simulink model "ship2021a"  (R2021a)
settings: Solver=VariableStepAuto  StartTime=0.0  StopTime=1500  RelTol=1e-3
undefined symbols (not defined in the file): D, Dn, M, surge_lambda, surge_omega_n, surge_zeta
libraries: mssSimulink x3, simulink x1
settings Model: Creator=simengangstad  LastModifiedBy=simengangstad

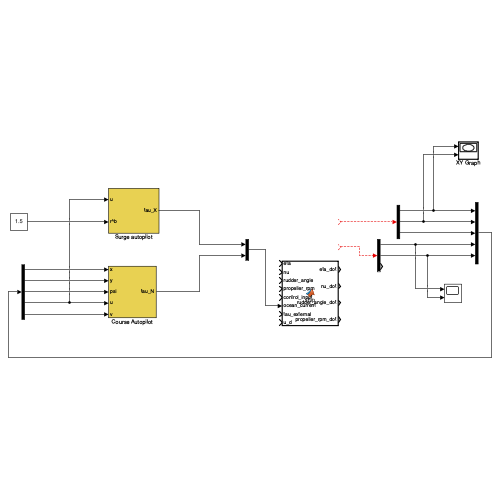
[thumbnail: Simulink's stored preview of the top-level diagram]
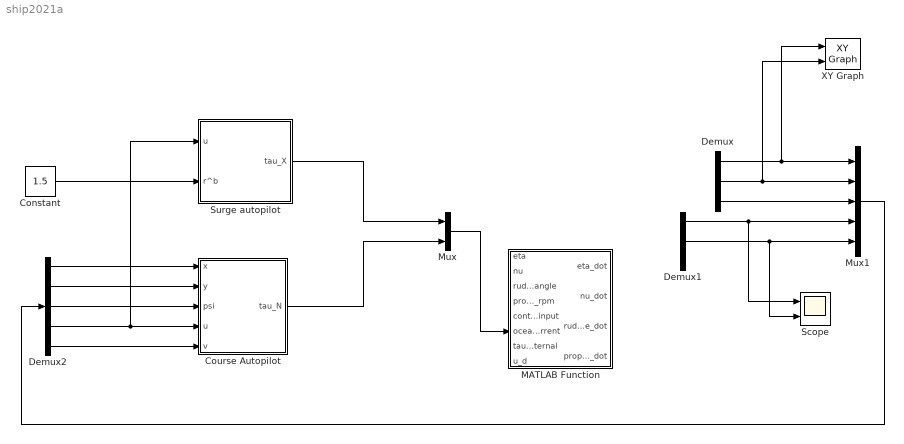
== system ship2021a ==
  Constant : Constant  Value=1.5
  Course Autopilot : Subsystem
  Demux : Demux  Outputs=3
  Demux1 : Demux  Outputs=3
  Demux2 : Demux  Outputs=5
  MATLAB Function : MATLAB Function  TreatAsAtomicUnit=on
  Mux : Mux  Inputs=2
  Mux1 : Mux  Inputs=5
  Scope : Scope  NumInputPorts=2
  Surge autopilot : Subsystem
  XY Graph : simulink/Sinks/XY Graph  xmin=-1  xmax=1  ymin=-1  ymax=1  st=-1
  wires:
  ? -> Demux1/1
  ? -> Demux/1
  Demux/2 -> XY Graph/2, Mux1/2
  Demux1/1 -> Scope/1, Mux1/4
  Constant/1 -> Surge autopilot/2(r^b)
  Surge autopilot/1(tau_X) -> Mux/1
  Demux/1 -> XY Graph/1, Mux1/1
  Demux/3 -> Mux1/3
  Demux1/2 -> Scope/2, Mux1/5
  Demux2/1 -> Course Autopilot/1(x)
  Demux2/2 -> Course Autopilot/2(y)
  Demux2/3 -> Course Autopilot/3(psi)
  Demux2/4 -> Surge autopilot/1(u), Course Autopilot/4(u)
  Demux2/5 -> Course Autopilot/5(v)
  Mux1/1 -> Demux2/1
  Course Autopilot/1(tau_N) -> Mux/2
  Mux/1 -> MATLAB Function/6(ocean_current)

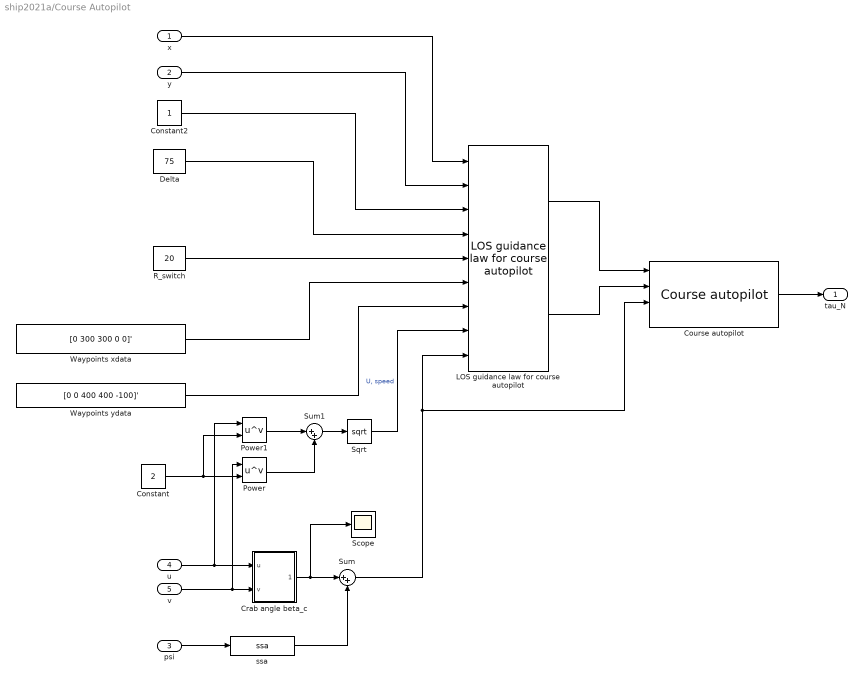
== system ship2021a/Course Autopilot ==
  x : Inport
  y : Inport  Port=2
  psi : Inport  Port=3
  u : Inport  Port=4
  v : Inport  Port=5
  Constant : Constant  Value=2
  Constant2 : Constant
  Course autopilot : mssSimulink/Control/Autopilots/Course autopilot  wn=yaw_omega_n  zeta=1  T_nomoto=yaw_T  m=M(3, 3)
  Crab angle beta_c : Subsystem
  Delta : Constant  Value=75
  LOS guidance law for course autopilot : mssSimulink/Guidance/LOS guidance law for course autopilot  SystemSampleTime=-1  VariantActivationTime=update diagram  Latency=0  AutoFrameSizeCalculation=off
  Power : Math  Operator=pow  SaturateOnIntegerOverflow=on
  Power1 : Math  Operator=pow  SaturateOnIntegerOverflow=on
  R_switch : Constant  Value=20
  Scope : Scope
  Sqrt : Sqrt  SaturateOnIntegerOverflow=on
  Sum : Sum  Inputs=|++
  Sum1 : Sum  Inputs=|++
  Waypoints xdata : Constant  Value=[0 300 300 0 0]'
  Waypoints ydata : Constant  Value=[0 0 400 400 -100]'
  "ssa   " : mssSimulink/Utilities/Math Operations/ssa  SystemSampleTime=-1  VariantActivationTime=update diagram  Latency=0  AutoFrameSizeCalculation=off
  tau_N : Outport
  wires:
  Sqrt/1 -> LOS guidance law for course autopilot/8  "U, speed"
  Course autopilot/1 -> tau_N/1
  x/1 -> LOS guidance law for course autopilot/1
  Delta/1 -> LOS guidance law for course autopilot/4
  y/1 -> LOS guidance law for course autopilot/2
  Sum/1 -> LOS guidance law for course autopilot/9, Course autopilot/3
  Constant2/1 -> LOS guidance law for course autopilot/3
  Waypoints xdata/1 -> LOS guidance law for course autopilot/6
  Waypoints ydata/1 -> LOS guidance law for course autopilot/7
  LOS guidance law for course autopilot/1 -> Course autopilot/1
  LOS guidance law for course autopilot/2 -> Course autopilot/2
  R_switch/1 -> LOS guidance law for course autopilot/5
  u/1 -> Crab angle beta_c/1(u), Power1/1
  v/1 -> Power/1, Crab angle beta_c/2(v)
  psi/1 -> "ssa   "/1
  Crab angle beta_c/1(beta_c) -> Scope/1, Sum/1
  "ssa   "/1 -> Sum/2
  Constant/1 -> Power1/2, Power/2
  Power1/1 -> Sum1/1
  Power/1 -> Sum1/2
  Sum1/1 -> Sqrt/1

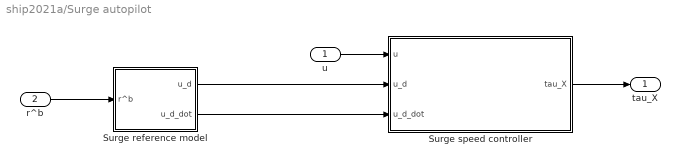
== system ship2021a/Surge autopilot ==
  u : Inport
  r^b : Inport  Port=2
  Surge reference model : Subsystem
  Surge speed controller : Subsystem
  tau_X : Outport
  wires:
  u/1 -> Surge speed controller/1(u)
  Surge reference model/1(u_d) -> Surge speed controller/2("u_d ")
  Surge speed controller/1(tau_X) -> tau_X/1
  Surge reference model/2(u_d_dot) -> Surge speed controller/3("u_d_dot ")
  r^b/1 -> Surge reference model/1(r^b)

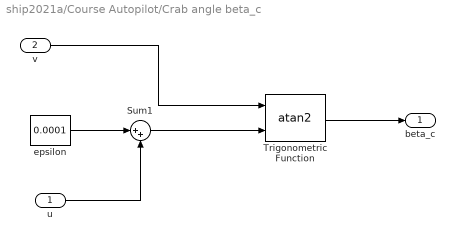
== system ship2021a/Course Autopilot/Crab angle beta_c ==
  u : Inport
  v : Inport  Port=2
  Sum1 : Sum  Inputs=|++  InputSameDT=on  SaturateOnIntegerOverflow=on  OutDataTypeStr=Inherit: Same as first input
  Trigonometric Function : Trigonometry  Operator=atan2
  epsilon : Constant  Value=0.0001
  beta_c : Outport
  wires:
  Trigonometric Function/1 -> beta_c/1
  v/1 -> Trigonometric Function/1
  Sum1/1 -> Trigonometric Function/2
  u/1 -> Sum1/2
  epsilon/1 -> Sum1/1

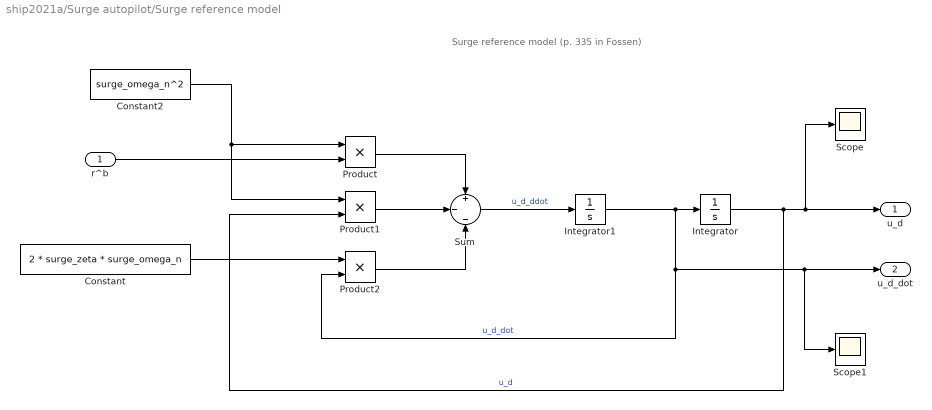
== system ship2021a/Surge autopilot/Surge reference model ==
  note: Surge reference model (p. 335 in Fossen)
  r^b : Inport
  Constant : Constant  Value=2 * surge_zeta * surge_omega_n
  Constant2 : Constant  Value=surge_omega_n^2
  Integrator : Integrator
  Integrator1 : Integrator
  Product : Product
  Product1 : Product
  Product2 : Product
  Scope : Scope
  Scope1 : Scope
  Sum : Sum  Inputs=+|-|-
  u_d : Outport
  u_d_dot : Outport  Port=2
  wires:
  r^b/1 -> Product/2
  Product2/1 -> Sum/3
  Product/1 -> Sum/1
  Constant/1 -> Product2/1
  Sum/1 -> Integrator1/1  "u_d_ddot"
  Constant2/1 -> Product/1, Product1/1
  Product1/1 -> Sum/2
  Integrator/1 -> Scope/1, u_d/1, Product1/2  "u_d"
  Integrator1/1 -> u_d_dot/1, Scope1/1, Product2/2, Integrator/1  "u_d_dot"

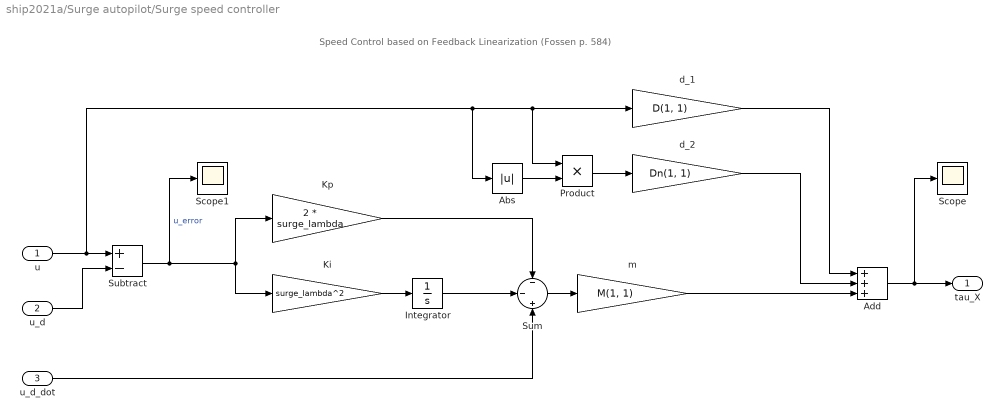
== system ship2021a/Surge autopilot/Surge speed controller ==
  note: Speed Control based on Feedback Linearization (Fossen p. 584)
  u : Inport
  "u_d " : Inport  Port=2
  "u_d_dot " : Inport  Port=3
  Abs : Abs
  Add : Sum  Inputs=+++
  Integrator : Integrator
  Ki : Gain  Gain=surge_lambda^2  SaturateOnIntegerOverflow=on  OutDataTypeStr=Inherit: Same as input  ParamDataTypeStr=Inherit: Same as input
  Kp : Gain  Gain=2 * surge_lambda  SaturateOnIntegerOverflow=on  OutDataTypeStr=Inherit: Same as input  ParamDataTypeStr=Inherit: Same as input
  Product : Product
  Scope : Scope
  Scope1 : Scope
  Subtract : Sum  Inputs=+-
  Sum : Sum  Inputs=-|-|+
  d_1 : Gain  Gain=D(1, 1)  SaturateOnIntegerOverflow=on  OutDataTypeStr=Inherit: Same as input  ParamDataTypeStr=Inherit: Same as input
  d_2 : Gain  Gain=Dn(1, 1)  SaturateOnIntegerOverflow=on  OutDataTypeStr=Inherit: Same as input  ParamDataTypeStr=Inherit: Same as input
  m : Gain  Gain=M(1, 1)  SaturateOnIntegerOverflow=on  OutDataTypeStr=Inherit: Same as input  ParamDataTypeStr=Inherit: Same as input
  tau_X : Outport
  wires:
  d_2/1 -> Add/2
  Product/1 -> d_2/1
  Ki/1 -> Integrator/1
  Sum/1 -> m/1
  Abs/1 -> Product/2
  Integrator/1 -> Sum/2
  u/1 -> Abs/1, Product/1, d_1/1, Subtract/1
  m/1 -> Add/3
  d_1/1 -> Add/1
  Add/1 -> Scope/1, tau_X/1
  Kp/1 -> Sum/1
  "u_d "/1 -> Subtract/2
  "u_d_dot "/1 -> Sum/3
  Subtract/1 -> Scope1/1, Ki/1, Kp/1  "u_error"

== matlab function ship2021a/MATLAB Function ==
  data: eta input; nu input; rudder_angle input; propeller_rpm input; control_input input; eta_dot output; nu_dot output; rudder_angle_dot output; propeller_rpm_dot output; ocean_current input; tau_external input; u_d input
function [eta_dot, nu_dot, rudder_angle_dot, propeller_rpm_dot] = ship(eta, nu, rudder_angle, propeller_rpm, control_input, ocean_current, tau_external, u_d)
%
% returns the time derivative of the state vector: 
% 
% eta   = [x y psi]
% nu    = [u v r]
% delta = actual rudder angle               (rad)
% n     = actual shaft velocity             (rpm)
% 
% The input vector is :
%
% u       = [ delta_c  n_c ]'  where
%
% delta_c = commanded rudder angle          (rad)
% n_c     = commanded shaft velocity        (rpm)
%
% The ocean current vector is: 
%
% nu_c    = [ u_c v_c 0 ]'  where
%
% uc = current velocity in surge            (m/s)
% vc = current velocity in sway             (m/s)
%
% The external environmental force vector is denoted by tau_ext


% Check of input and state dimensions
if length(x) ~= 8
    error('x-vector must have dimension 8 !');
end

if length(u) ~= 2
    error('u-vector must have dimension 2 !');
end

% Dimensional states and input
delta_c = u(1); 
n_c     = u(2);

nu      = x(1:3);
eta     = x(4:6);
delta   = x(7);
n       = x(8); 


nu_r = nu - nu_c;       % Relative velocity
uc = nu_c(1);
vc = nu_c(2);


% Parameters 
m   = 17.0677e6;         % Total mass (kg)
Iz  = 2.1732e10;         % Yaw moment of inertia (kg m^2)
xg  = -3.7;              % CG x-ccordinate (m)
L   = 161;               % length (m)
B   = 21.8;              % beam (m)
T   = 8.9;               % draft (m)
KT  = 0.6367;            % propeller coefficient (-)
KQ  = 0.1390;
Dia = 3.3;               % propeller diameter (m)
rho = 1025;              % density of water (m/s^3)

% Propeller parameters
I_m = 100000;            % Inertia of the rotating parts including the propeller
                         % and added inertia of the water (kgm^2)
T_m = 10;                

% Rudder limitations
delta_max  = 40 * pi/180;        % max rudder angle      (rad)
Ddelta_max = 5  * pi/180;        % max rudder derivative (rad/s)

% Added mass matrix
Xudot = -8.9830e5;
Yvdot = -5.1996e6;
Yrdot =  9.3677e5;
Nvdot =  Yrdot;
Nrdot = -2.4283e10;
MA = -[ Xudot 0 0; 0 Yvdot Yrdot; 0 Nvdot Nrdot ];   % Added mass matrix

% Rigid-body mass matrix
MRB = [ m 0      0 
        0 m      m * xg
        0 m * xg Iz ];        
Minv = inv(MRB + MA);       

% Rudder coefficients
b = 2;
AR = 8;
CB = 0.8;

lambda = b^2 / AR;
tR = 0.45 - 0.28*CB;
CN = 6.13 * lambda / (lambda + 2.25);
aH = 0.75;
xH = -0.4 * L;
xR = -0.5 * L;

% Input matrix
t_thr = 0.05;                                        % Thrust deduction number
X_delta2 = 0.5 * (1 - tR) * rho * AR * CN;           % Rudder coefficients
Y_delta = 0.25 * (1 + aH) * rho * AR * CN; 
N_delta = 0.25 * (xR + aH * xH) * rho * AR * CN;   

Bi = @(u_r,delta) [ (1-t_thr)  -u_r^2 * X_delta2 * delta
                        0      -u_r^2 * Y_delta
                        0      -u_r^2 * N_delta            ];
    
% State-dependent time-varying matrices

% Restoring force for rigid-body
CRB = m * nu_r(3) * [ 0 -1 -xg 
                      1  0  0 
                      xg 0  0  ];         

% Restoring force for added mass 
CA = [0 0 Yvdot * nu_r(2) + Yrdot * nu_r(3); 
      0 0 -Xudot * nu_r(1); 
      -Yvdot * nu_r(2) - Yrdot * nu_r(3) Xudot * nu_r(1) 0];    

% Linear damping
T1 = 20; T2 = 20; T6 = 10;      % Natural Period for Surge, Sway and Yaw (s)
Xu = -(m-Xudot) / T1;
Yv = -(m-Yvdot) / T2;
Nr = -(Iz-Nrdot) / T6;
D = -diag([Xu Yv Nr]); 

% Nonlinear surge damping
eps = 0.001;
CR = 0;
k = 0.1;
S = B*L + 2*T*(B+L);
v = 1e-6;
Rn = L / v * abs(nu_r(1));
Cf = 0.075 / (log10(Rn) - 2 + eps)^2 + CR;
Xns = -0.5 * rho * S * (1+k) * Cf * abs(nu_r(1)) * nu_r(1);

% Nonlinear cross-flow drag
Cd_2d = Hoerner(B,T);
dx = L/10;
Ycf = 0; Ncf = 0;
for xL = -L/2:dx:L/2
    Ucf = abs(nu_r(2) + xL * nu_r(3)) * (nu_r(2) + xL * nu_r(3));
    Ycf = Ycf - 0.5 * rho * T * Cd_2d * Ucf * dx;
    Ncf = Ncf - 0.5 * rho * T * Cd_2d * xL * Ucf * dx;
end
d = -[Xns Ycf Ncf]';

% Thrust
thr = rho * Dia^4 * KT * abs(n) * n;

% Ship dynamics
R = Rzyx(0, 0, eta(3));
u = [ thr delta ]';
tau = Bi(nu_r(1), delta) * u;

nu_dot = [nu(3) * vc -nu(3) * uc 0]' + Minv * (tau_ext + tau - (CRB + CA + D) * nu_r - d);
eta_dot = R * nu;    

% Rudder saturation and dynamics
if abs(delta_c) >= delta_max
    delta_c = sign(delta_c)*delta_max;
end

delta_dot = delta_c - delta;
if abs(delta_dot) >= Ddelta_max
    delta_dot = sign(delta_dot)*Ddelta_max;
end    

% Propeller dynamics
t = 0.1;
T_d = Xu * u_d / (t - 1);
K_ff_u = sign(T_d) * sqrt(abs(T_d) / (rho * Dia^4 * KT));  % Feed foreward on u
n_c = n_c + K_ff_u;                                        % propeller speed (rps)

Q_d =  rho * Dia^5 * KQ * abs(n_c) * n_c;
Q_m = 1/(1+T_m) * Q_d;
K_ff_n = rho * Dia^5 * KQ * abs(n) * n;         % Feed foreward on n
K_p_n = 1;
Q = K_p_n * (n - n_c) + K_ff_n;                 % Feedback and foreward (on n)

n_dot = (Q_m - Q)/I_m;                          % Assume Q_f = 0

xdot = [nu_dot' eta_dot' delta_dot n_dot]';
u = [delta_c n_c]';
end
